simulink model "ES102A_PolarityCfg"
settings: Solver=ode45  StartTime=0.0  StopTime=10.0  RelTol=1e-3
undefined symbols (not defined in the file or in its folder): sigbuilder_block
libraries: simulink x29
(part 4 of 4)

== system ES102A_PolarityCfg/PolarityCfg/PolarityCfgInit1/SysPolarity/If Action Subsystem1 ==
  Action Port : ActionPort  ActionType=else
  Constant : Constant  Value=-1
  Copyright1 : Subsystem  Description=|  mask(Copyright Information){none=on}
      | Copyright info block.                                               
      |                                                                     
      | Place copyright information at the top of every subsystem in design.
      mask prompts: none "No parameters"
      mask help: Place copyright information at the top of every subsystem in design.
      mask Display:
      | NxtrConf = 'Nexteer Confidential';
      | 
      | sys = bdroot; %handle for the current model ("system")
      | first = get_param(sys,'Created');
      | if(isempty(first))
      |     first = datestr(now,'yyyy');
      | else
      |     first = first(end-3:end);  %year is last four digits
      | end
      | 
      | last = get_param(sys,'LastModifiedDate');
      | if isempty(last)
      |     last = datestr(now,'yyyy');
      | else
      |     last = last(end-3:end);
      | end
      | 
      | if strcmp(first,last)
      |     fprintf('%s\nCopyright  %s Nexteer',NxtrConf,first);
      | else
      |     fprintf('%s\n%s%s-%s Nexteer',NxtrConf,char(169),first,last);
      | end
  Out1 : Outport  InitialOutput=-1
  wires:
  Constant/1 -> Out1/1

== system ES102A_PolarityCfg/PolarityCfg/PolarityCfgInit1/SysPolarity/If Action Subsystem2 ==
  Action Port : ActionPort  ActionType=then
  Constant : Constant
  Copyright1 : Subsystem  Description=|  mask(Copyright Information){none=on}
      | Copyright info block.                                               
      |                                                                     
      | Place copyright information at the top of every subsystem in design.
      mask prompts: none "No parameters"
      mask help: Place copyright information at the top of every subsystem in design.
      mask Display:
      | NxtrConf = 'Nexteer Confidential';
      | 
      | sys = bdroot; %handle for the current model ("system")
      | first = get_param(sys,'Created');
      | if(isempty(first))
      |     first = datestr(now,'yyyy');
      | else
      |     first = first(end-3:end);  %year is last four digits
      | end
      | 
      | last = get_param(sys,'LastModifiedDate');
      | if isempty(last)
      |     last = datestr(now,'yyyy');
      | else
      |     last = last(end-3:end);
      | end
      | 
      | if strcmp(first,last)
      |     fprintf('%s\nCopyright  %s Nexteer',NxtrConf,first);
      | else
      |     fprintf('%s\n%s%s-%s Nexteer',NxtrConf,char(169),first,last);
      | end
  Out1 : Outport  InitialOutput=1
  wires:
  Constant/1 -> Out1/1

== system ES102A_PolarityCfg/PolarityCfg/PolarityCfgInit1/SysPolarity/If Action Subsystem3 ==
  Action Port : ActionPort  ActionType=else
  Constant : Constant  Value=-1
  Copyright1 : Subsystem  Description=|  mask(Copyright Information){none=on}
      | Copyright info block.                                               
      |                                                                     
      | Place copyright information at the top of every subsystem in design.
      mask prompts: none "No parameters"
      mask help: Place copyright information at the top of every subsystem in design.
      mask Display:
      | NxtrConf = 'Nexteer Confidential';
      | 
      | sys = bdroot; %handle for the current model ("system")
      | first = get_param(sys,'Created');
      | if(isempty(first))
      |     first = datestr(now,'yyyy');
      | else
      |     first = first(end-3:end);  %year is last four digits
      | end
      | 
      | last = get_param(sys,'LastModifiedDate');
      | if isempty(last)
      |     last = datestr(now,'yyyy');
      | else
      |     last = last(end-3:end);
      | end
      | 
      | if strcmp(first,last)
      |     fprintf('%s\nCopyright  %s Nexteer',NxtrConf,first);
      | else
      |     fprintf('%s\n%s%s-%s Nexteer',NxtrConf,char(169),first,last);
      | end
  Out1 : Outport  InitialOutput=-1
  wires:
  Constant/1 -> Out1/1

== system ES102A_PolarityCfg/PolarityCfg/PolarityCfgInit1/HwAgPolarity/If Action Subsystem/Copyright1 ==

== system ES102A_PolarityCfg/PolarityCfg/PolarityCfgInit1/HwAgPolarity/If Action Subsystem1/Copyright1 ==

== system ES102A_PolarityCfg/PolarityCfg/PolarityCfgInit1/HwAgPolarity/If Action Subsystem10/Copyright1 ==

== system ES102A_PolarityCfg/PolarityCfg/PolarityCfgInit1/HwAgPolarity/If Action Subsystem11/Copyright1 ==

== system ES102A_PolarityCfg/PolarityCfg/PolarityCfgInit1/HwAgPolarity/If Action Subsystem12/Copyright1 ==

== system ES102A_PolarityCfg/PolarityCfg/PolarityCfgInit1/HwAgPolarity/If Action Subsystem13/Copyright1 ==

== system ES102A_PolarityCfg/PolarityCfg/PolarityCfgInit1/HwAgPolarity/If Action Subsystem14/Copyright1 ==

== system ES102A_PolarityCfg/PolarityCfg/PolarityCfgInit1/HwAgPolarity/If Action Subsystem15/Copyright1 ==

== system ES102A_PolarityCfg/PolarityCfg/PolarityCfgInit1/HwAgPolarity/If Action Subsystem2/Copyright1 ==

== system ES102A_PolarityCfg/PolarityCfg/PolarityCfgInit1/HwAgPolarity/If Action Subsystem3/Copyright1 ==

== system ES102A_PolarityCfg/PolarityCfg/PolarityCfgInit1/HwAgPolarity/If Action Subsystem4/Copyright1 ==

== system ES102A_PolarityCfg/PolarityCfg/PolarityCfgInit1/HwAgPolarity/If Action Subsystem5/Copyright1 ==

== system ES102A_PolarityCfg/PolarityCfg/PolarityCfgInit1/HwAgPolarity/If Action Subsystem6/Copyright1 ==

== system ES102A_PolarityCfg/PolarityCfg/PolarityCfgInit1/HwAgPolarity/If Action Subsystem7/Copyright1 ==

== system ES102A_PolarityCfg/PolarityCfg/PolarityCfgInit1/HwAgPolarity/If Action Subsystem8/Copyright1 ==

== system ES102A_PolarityCfg/PolarityCfg/PolarityCfgInit1/HwAgPolarity/If Action Subsystem9/Copyright1 ==

== system ES102A_PolarityCfg/PolarityCfg/PolarityCfgInit1/HwTqPolarity/If Action Subsystem/Copyright1 ==

== system ES102A_PolarityCfg/PolarityCfg/PolarityCfgInit1/HwTqPolarity/If Action Subsystem1/Copyright1 ==

== system ES102A_PolarityCfg/PolarityCfg/PolarityCfgInit1/HwTqPolarity/If Action Subsystem10/Copyright1 ==

== system ES102A_PolarityCfg/PolarityCfg/PolarityCfgInit1/HwTqPolarity/If Action Subsystem11/Copyright1 ==

== system ES102A_PolarityCfg/PolarityCfg/PolarityCfgInit1/HwTqPolarity/If Action Subsystem12/Copyright1 ==

== system ES102A_PolarityCfg/PolarityCfg/PolarityCfgInit1/HwTqPolarity/If Action Subsystem13/Copyright1 ==

== system ES102A_PolarityCfg/PolarityCfg/PolarityCfgInit1/HwTqPolarity/If Action Subsystem14/Copyright1 ==

== system ES102A_PolarityCfg/PolarityCfg/PolarityCfgInit1/HwTqPolarity/If Action Subsystem15/Copyright1 ==

== system ES102A_PolarityCfg/PolarityCfg/PolarityCfgInit1/HwTqPolarity/If Action Subsystem2/Copyright1 ==

== system ES102A_PolarityCfg/PolarityCfg/PolarityCfgInit1/HwTqPolarity/If Action Subsystem3/Copyright1 ==

== system ES102A_PolarityCfg/PolarityCfg/PolarityCfgInit1/HwTqPolarity/If Action Subsystem4/Copyright1 ==

== system ES102A_PolarityCfg/PolarityCfg/PolarityCfgInit1/HwTqPolarity/If Action Subsystem5/Copyright1 ==

== system ES102A_PolarityCfg/PolarityCfg/PolarityCfgInit1/HwTqPolarity/If Action Subsystem6/Copyright1 ==

== system ES102A_PolarityCfg/PolarityCfg/PolarityCfgInit1/HwTqPolarity/If Action Subsystem7/Copyright1 ==

== system ES102A_PolarityCfg/PolarityCfg/PolarityCfgInit1/HwTqPolarity/If Action Subsystem8/Copyright1 ==

== system ES102A_PolarityCfg/PolarityCfg/PolarityCfgInit1/HwTqPolarity/If Action Subsystem9/Copyright1 ==

== system ES102A_PolarityCfg/PolarityCfg/PolarityCfgInit1/MotAgMeclPolarity/If Action Subsystem/Copyright1 ==

== system ES102A_PolarityCfg/PolarityCfg/PolarityCfgInit1/MotAgMeclPolarity/If Action Subsystem1/Copyright1 ==

== system ES102A_PolarityCfg/PolarityCfg/PolarityCfgInit1/MotAgMeclPolarity/If Action Subsystem10/Copyright1 ==

== system ES102A_PolarityCfg/PolarityCfg/PolarityCfgInit1/MotAgMeclPolarity/If Action Subsystem11/Copyright1 ==

== system ES102A_PolarityCfg/PolarityCfg/PolarityCfgInit1/MotAgMeclPolarity/If Action Subsystem12/Copyright1 ==

== system ES102A_PolarityCfg/PolarityCfg/PolarityCfgInit1/MotAgMeclPolarity/If Action Subsystem13/Copyright1 ==

== system ES102A_PolarityCfg/PolarityCfg/PolarityCfgInit1/MotAgMeclPolarity/If Action Subsystem14/Copyright1 ==

== system ES102A_PolarityCfg/PolarityCfg/PolarityCfgInit1/MotAgMeclPolarity/If Action Subsystem15/Copyright1 ==

== system ES102A_PolarityCfg/PolarityCfg/PolarityCfgInit1/MotAgMeclPolarity/If Action Subsystem2/Copyright1 ==

== system ES102A_PolarityCfg/PolarityCfg/PolarityCfgInit1/MotAgMeclPolarity/If Action Subsystem3/Copyright1 ==

== system ES102A_PolarityCfg/PolarityCfg/PolarityCfgInit1/MotAgMeclPolarity/If Action Subsystem4/Copyright1 ==

== system ES102A_PolarityCfg/PolarityCfg/PolarityCfgInit1/MotAgMeclPolarity/If Action Subsystem5/Copyright1 ==

== system ES102A_PolarityCfg/PolarityCfg/PolarityCfgInit1/MotAgMeclPolarity/If Action Subsystem6/Copyright1 ==

== system ES102A_PolarityCfg/PolarityCfg/PolarityCfgInit1/MotAgMeclPolarity/If Action Subsystem7/Copyright1 ==

== system ES102A_PolarityCfg/PolarityCfg/PolarityCfgInit1/MotAgMeclPolarity/If Action Subsystem8/Copyright1 ==

== system ES102A_PolarityCfg/PolarityCfg/PolarityCfgInit1/SysPolarity/If Action Subsystem/Copyright1 ==

== system ES102A_PolarityCfg/PolarityCfg/PolarityCfgInit1/SysPolarity/If Action Subsystem1/Copyright1 ==

== system ES102A_PolarityCfg/PolarityCfg/PolarityCfgInit1/SysPolarity/If Action Subsystem2/Copyright1 ==

== system ES102A_PolarityCfg/PolarityCfg/PolarityCfgInit1/SysPolarity/If Action Subsystem3/Copyright1 ==
